simulink model "FOC_RL"  (R2023b)
settings: Solver=VariableStepAuto  StartTime=0.0  StopTime=30  RelTol=1e-3
InitFcn:
  | Resistencia = 0.679;
  | Inductancia = 0.01;
undefined symbols (not defined in the file): angulo, frac_polar, fuerza, magnitude
libraries: eeTransforms x3, slpidlib x3
settings Model: Creator=USUARIO  LastModifiedBy=USUARIO

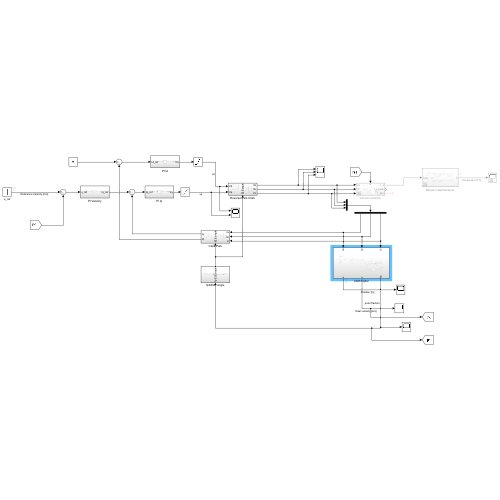
[thumbnail: Simulink's stored preview of the top-level diagram]
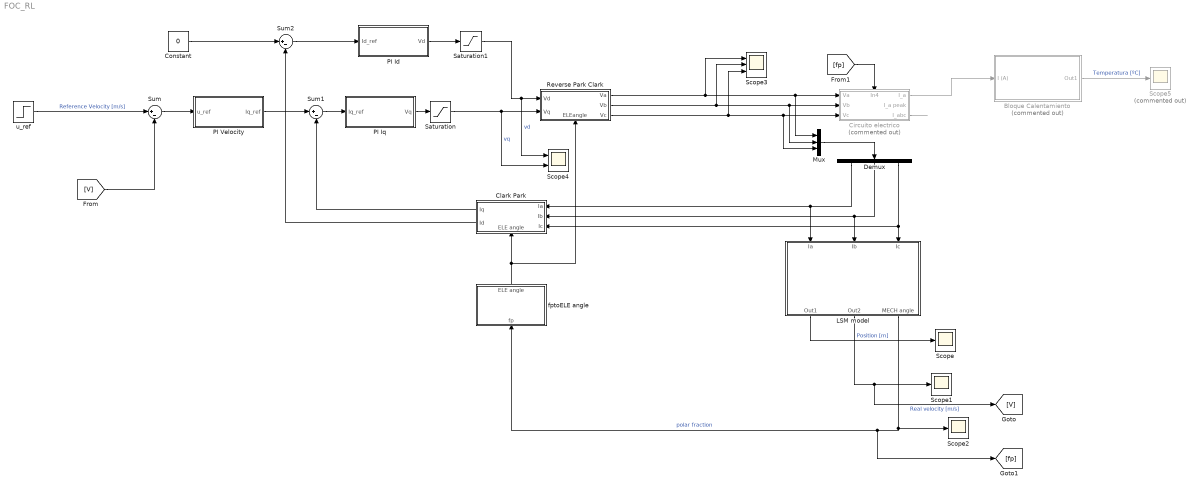
== system FOC_RL ==
  Bloque Calentamiento : Subsystem  Commented=on
  Circuito electrico : Subsystem  Commented=on
      settings: PortSchema="{\"entries\":[{\"content\":{\"sides\":[{\"content\":{\"connectorIds\":[\"In1\",\"In2\",\"In3\"]},\"type\":\"ConnectorPlacement.EquallySpacedRectSide\",\"uuid\":\"3f81a6db-fb69-453a-a09a-736cf4e6fbdf\"},{\"content\":{\"connectorIds\":[\"Out1\",\"Out2\",\"Out3\"],\"side\":\"RIGHT\"},\"type\":\"ConnectorPlacement.EquallySpacedRectSide\",\"uuid\":\"28f19065-0fce-4caf-9d5e-808d35e6acc4\"},{\"content\":{\"connectorIds\":[\"In4\"],\"side\":\"TOP\"},\"type\":\"ConnectorPlacement.EquallySpacedRectSide\",\"uuid\":\"0f0f3d94-64b2-4ad8-85c5-3a76de2037a2\"}]},\"type\":\"ConnectorPlacement.EquallySpacedConnector\",\"uuid\":\"ca84a14e-6f4b-4b2e-8a9f-b6683e76143b\"}],\"packageUris\":[\"http://schema.mathworks.com/mf0/Connector/R2020b\"],\"version\":\"1.0\"}"
  Clark Park : Subsystem
      settings: PortSchema="{\"entries\":[{\"content\":{\"sides\":[{\"content\":{\"connectorIds\":[\"Out1\",\"Out2\"]},\"type\":\"ConnectorPlacement.EquallySpacedRectSide\",\"uuid\":\"b73a0972-bf68-45ae-9239-d3343df02446\"},{\"content\":{\"connectorIds\":[\"In2\",\"In3\",\"In4\"],\"side\":\"RIGHT\"},\"type\":\"ConnectorPlacement.EquallySpacedRectSide\",\"uuid\":\"fec89271-c2ef-4885-992a-4c0db260d6e2\"},{\"content\":{\"side\":\"TOP\"},\"type\":\"ConnectorPlacement.EquallySpacedRectSide\",\"uuid\":\"51dbb3d3-34a9-43d7-9c98-9fa2f2011719\"},{\"content\":{\"connectorIds\":[\"In1\"],\"side\":\"BOTTOM\"},\"type\":\"ConnectorPlacement.EquallySpacedRectSide\",\"uuid\":\"eab6f42e-44ed-4b27-921c-43f03788cacc\"}]},\"type\":\"ConnectorPlacement.EquallySpacedConnector\",\"uuid\":\"a64495c7-a005-4dee-b109-5230f9247adc\"}],\"packageUris\":[\"http://schema.mathworks.com/mf0/Connector/R2020b\"],\"version\":\"1.0\"}"
  Constant : Constant  Value=0
  Demux : Demux  Outputs=3
  LSM model : Subsystem
      settings: PortSchema="{\"entries\":[{\"content\":{\"sides\":[{\"content\":{},\"type\":\"ConnectorPlacement.EquallySpacedRectSide\",\"uuid\":\"cac53d69-c428-44dc-bdf5-c688872b0596\"},{\"content\":{\"side\":\"RIGHT\"},\"type\":\"ConnectorPlacement.EquallySpacedRectSide\",\"uuid\":\"eab58244-5d35-448a-9540-885c93543b87\"},{\"content\":{\"connectorIds\":[\"In1\",\"In2\",\"In3\"],\"side\":\"TOP\"},\"type\":\"ConnectorPlacement.EquallySpacedRectSide\",\"uuid\":\"c64ce138-6960-4dd5-9e90-e1ffecc69b70\"},{\"content\":{\"connectorIds\":[\"Out1\",\"Out2\",\"Out3\"],\"side\":\"BOTTOM\"},\"type\":\"ConnectorPlacement.EquallySpacedRectSide\",\"uuid\":\"eda83129-b662-4da7-9603-68b1882420cc\"}]},\"type\":\"ConnectorPlacement.EquallySpacedConnector\",\"uuid\":\"82b650b8-86c6-4f03-ba07-634d14e4b94d\"}],\"packageUris\":[\"http://schema.mathworks.com/mf0/Connector/R2020b\"],\"version\":\"1.0\"}"
  Mux : Mux  Inputs=3
  PI Id : Subsystem
  PI Iq : Subsystem
  PI Velocity : Subsystem
  Reverse Park Clark : Subsystem
      settings: PortSchema="{\"entries\":[{\"content\":{\"sides\":[{\"content\":{\"connectorIds\":[\"In1\",\"In2\"]},\"type\":\"ConnectorPlacement.EquallySpacedRectSide\",\"uuid\":\"bb4b1d20-48ba-4b2f-b253-a250226ab501\"},{\"content\":{\"connectorIds\":[\"Out1\",\"Out2\",\"Out3\"],\"side\":\"RIGHT\"},\"type\":\"ConnectorPlacement.EquallySpacedRectSide\",\"uuid\":\"4768cfae-b67e-4820-9de3-2f5fe637e53a\"},{\"content\":{\"side\":\"TOP\"},\"type\":\"ConnectorPlacement.EquallySpacedRectSide\",\"uuid\":\"af639b0a-05db-45f8-bbbc-8f88455894ca\"},{\"content\":{\"connectorIds\":[\"In3\"],\"side\":\"BOTTOM\"},\"type\":\"ConnectorPlacement.EquallySpacedRectSide\",\"uuid\":\"149993ad-8fc7-43c9-baef-e4c40b0fb2ea\"}]},\"type\":\"ConnectorPlacement.EquallySpacedConnector\",\"uuid\":\"6dc62ad4-a38d-4494-a0f6-179f186f788d\"}],\"packageUris\":[\"http://schema.mathworks.com/mf0/Connector/R2020b\"],\"version\":\"1.0\"}"
  Saturation : Saturate  UpperLimit=100  LowerLimit=-100
  Saturation1 : Saturate  UpperLimit=100  LowerLimit=-100
  Scope : Scope
  Scope1 : Scope
  Scope2 : Scope
  Scope3 : Scope  NumInputPorts=3
  Scope4 : Scope  NumInputPorts=2
  Scope5 : Scope  Commented=on
  Sum : Sum  Inputs=|+-
  Sum1 : Sum  Inputs=|+-
  Sum2 : Sum  Inputs=|+-
  fptoELE angle : Subsystem
      settings: PortSchema="{\"entries\":[{\"content\":{\"sides\":[{\"content\":{},\"type\":\"ConnectorPlacement.EquallySpacedRectSide\",\"uuid\":\"b73a0972-bf68-45ae-9239-d3343df02446\"},{\"content\":{\"side\":\"RIGHT\"},\"type\":\"ConnectorPlacement.EquallySpacedRectSide\",\"uuid\":\"fec89271-c2ef-4885-992a-4c0db260d6e2\"},{\"content\":{\"connectorIds\":[\"Out1\"],\"side\":\"TOP\"},\"type\":\"ConnectorPlacement.EquallySpacedRectSide\",\"uuid\":\"51dbb3d3-34a9-43d7-9c98-9fa2f2011719\"},{\"content\":{\"connectorIds\":[\"In1\"],\"side\":\"BOTTOM\"},\"type\":\"ConnectorPlacement.EquallySpacedRectSide\",\"uuid\":\"4816d69c-9e54-4057-b439-390caef350ee\"}]},\"type\":\"ConnectorPlacement.EquallySpacedConnector\",\"uuid\":\"a64495c7-a005-4dee-b109-5230f9247adc\"}],\"packageUris\":[\"http://schema.mathworks.com/mf0/Connector/R2020b\"],\"version\":\"1.0\"}"
  u_ref : Step  Before=0.001  After=2  SampleTime=0
  wires:
  Constant/1 -> Sum2/1
  LSM model/3(MECH angle) -> [fp], fptoELE angle/1(fp), Scope2/1  "polar fraction"
  Clark Park/2(Id) -> Sum2/2
  Sum/1 -> PI Velocity/1(u_ref)
  fptoELE angle/1(ELE angle) -> Reverse Park Clark/3(ELEangle), Clark Park/1(ELE angle)
  Clark Park/1(Iq) -> Sum1/2
  PI Iq/1(Vq) -> Saturation/1
  Sum2/1 -> PI Id/1(Id_ref)
  Reverse Park Clark/3(Vc) -> Scope3/3, Mux/3, Circuito electrico/3(Vc)
  u_ref/1 -> Sum/1  "Reference Velocity [m/s]"
  Reverse Park Clark/2(Vb) -> Scope3/2, Mux/2, Circuito electrico/2(Vb)
  PI Id/1(Vd) -> Saturation1/1
  Reverse Park Clark/1(Va) -> Scope3/1, Mux/1, Circuito electrico/1(Va)
  Sum1/1 -> PI Iq/1(Iq_ref)
  LSM model/1(Out1) -> Scope/1  "Position [m]"
  LSM model/2(Out2) -> [V], Scope1/1  "Real velocity [m/s]"
  Saturation/1 -> Scope4/2, Reverse Park Clark/2(Vq)  "vq"
  Saturation1/1 -> Reverse Park Clark/1(Vd), Scope4/1  "vd"
  PI Velocity/1(Iq_ref) -> Sum1/1
  [V] -> Sum/2
  Bloque Calentamiento/1(Out1) -> Scope5/1  "Temperatura [ºC]"
  [fp] -> Circuito electrico/4(In4)
  Circuito electrico/3(I_abc) -> ?
  Circuito electrico/1(I_a) -> Bloque Calentamiento/1(I (A))
  Mux/1 -> Demux/1
  Demux/1 -> Clark Park/2(Ia), LSM model/1(Ia)
  Demux/2 -> Clark Park/3(Ib), LSM model/2(Ib)
  Demux/3 -> Clark Park/4(Ic), LSM model/3(Ic)

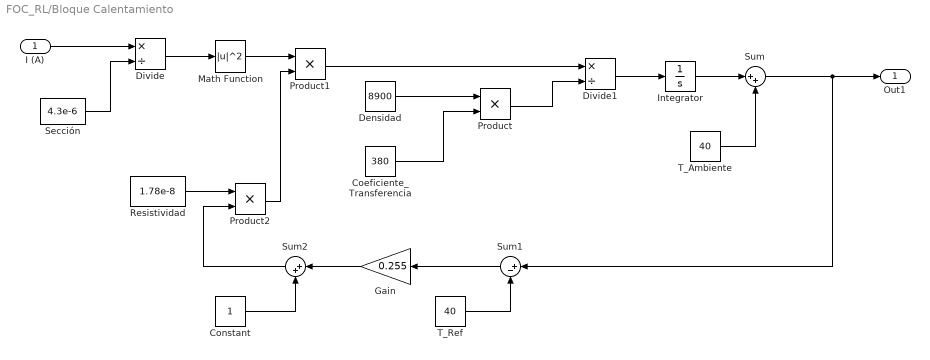
== system FOC_RL/Bloque Calentamiento ==
  I (A) : Inport
  Coeficiente_Transferencia : Constant  Value=380
  Constant : Constant
  Densidad : Constant  Value=8900
  Divide : Product  Inputs=*/
  Divide1 : Product  Inputs=*/
  Gain : Gain  Gain=0.255
  Integrator : Integrator
  Math Function : Math  Operator=magnitude^2
  Product : Product
  Product1 : Product
  Product2 : Product
  Resistividad : Constant  Value=1.78e-8
  Sección : Constant  Value=4.3e-6
  Sum : Sum  Inputs=|++
  Sum1 : Sum  Inputs=|+-
  Sum2 : Sum  Inputs=|++
  T_Ambiente : Constant  Value=40
  T_Ref : Constant  Value=40
  Out1 : Outport
  wires:
  I (A)/1 -> Divide/1
  Sección/1 -> Divide/2
  Divide/1 -> Math Function/1
  Densidad/1 -> Product/1
  Coeficiente_Transferencia/1 -> Product/2
  Product/1 -> Divide1/2
  Divide1/1 -> Integrator/1
  Math Function/1 -> Product1/1
  Product1/1 -> Divide1/1
  Resistividad/1 -> Product2/1
  Product2/1 -> Product1/2
  Integrator/1 -> Sum/1
  Sum/1 -> Sum1/1, Out1/1
  T_Ambiente/1 -> Sum/2
  Sum1/1 -> Gain/1
  T_Ref/1 -> Sum1/2
  Gain/1 -> Sum2/1
  Constant/1 -> Sum2/2
  Sum2/1 -> Product2/2

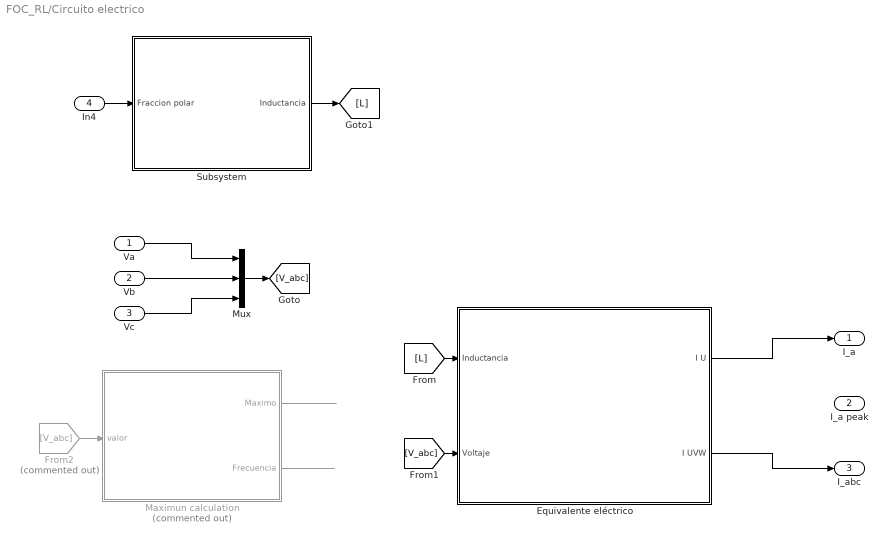
== system FOC_RL/Circuito electrico ==
  Va : Inport
  Vb : Inport  Port=2
  Vc : Inport  Port=3
  In4 : Inport  Port=4
  Equivalente eléctrico : Subsystem
  From2 : From  Commented=on  GotoTag=V_abc
  Maximun calculation : Subsystem  Commented=on
  Mux : Mux  Inputs=3
  Subsystem : Subsystem
  I_a : Outport
  I_a peak : Outport  Port=2
  I_abc : Outport  Port=3
  wires:
  Vc/1 -> Mux/3
  Vb/1 -> Mux/2
  Va/1 -> Mux/1
  Maximun calculation/2(Frecuencia) -> ?
  Maximun calculation/1(Maximo) -> ?
  Equivalente eléctrico/1(I U) -> I_a/1
  ? -> I_a peak/1
  Equivalente eléctrico/2(I UVW) -> I_abc/1
  Mux/1 -> [V_abc]
  Subsystem/1(Inductancia) -> [L]
  From2/1 -> Maximun calculation/1(valor)
  [V_abc] -> Equivalente eléctrico/2(Voltaje)
  [L] -> Equivalente eléctrico/1(Inductancia)
  In4/1 -> Subsystem/1(Fraccion polar)

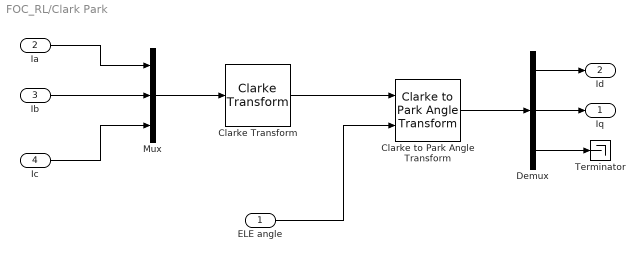
== system FOC_RL/Clark Park ==
  ELE angle : Inport
  Ia : Inport  Port=2
  Ib : Inport  Port=3
  Ic : Inport  Port=4
  Clarke Transform : eeTransforms/Clarke Transform  PowerInvariant=off
      settings: LibrarySourceBlock=|
      | ee_sl_lib/Mathematical
      | Transforms/Clarke Transform
  Clarke to Park Angle Transform : eeTransforms/Clarke to Park Angle Transform  AxisAlignment=Q-axis
      settings: LibrarySourceBlock=|
      | ee_sl_lib/Mathematical
      | Transforms/Clarke to Park
      | Angle Transform
  Demux : Demux  Outputs=3
  Mux : Mux  Inputs=3
  Terminator : Terminator
  Iq : Outport
  Id : Outport  Port=2
  wires:
  Ia/1 -> Mux/1
  Ib/1 -> Mux/2
  Ic/1 -> Mux/3
  Mux/1 -> Clarke Transform/1
  Clarke Transform/1 -> Clarke to Park Angle Transform/1
  ELE angle/1 -> Clarke to Park Angle Transform/2
  Clarke to Park Angle Transform/1 -> Demux/1
  Demux/1 -> Id/1
  Demux/2 -> Iq/1
  Demux/3 -> Terminator/1

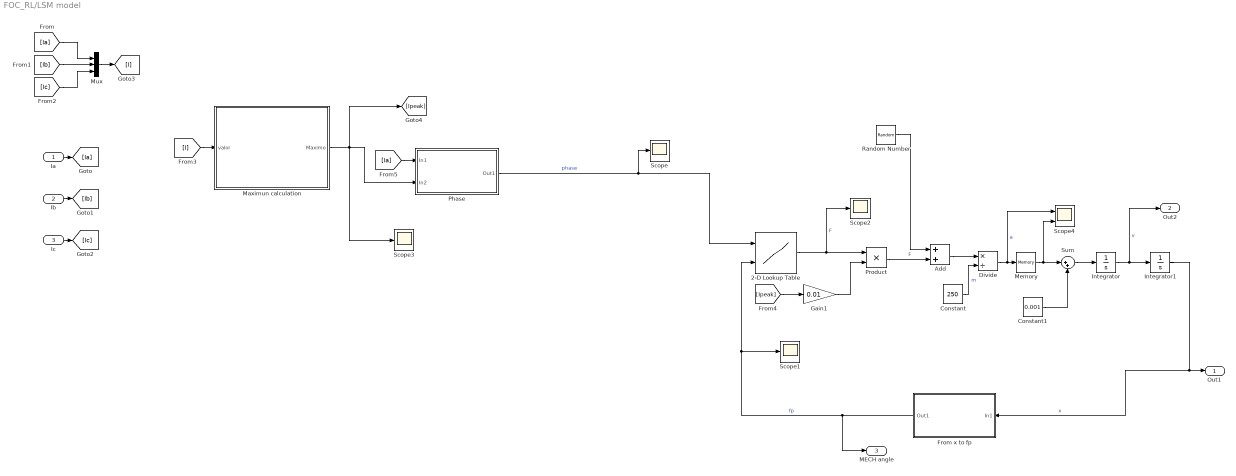
== system FOC_RL/LSM model ==
  Ia : Inport
  Ib : Inport  Port=2
  Ic : Inport  Port=3
  2-D Lookup Table : Lookup_n-D  BreakpointsForDimension1=angulo  BreakpointsForDimension2=frac_polar  Table=fuerza  InternalRulePriority=Speed  RndMeth=Simplest
      settings: InputPortMap=u0,u1
  Add : Sum
  Constant : Constant  Value=250
  Constant1 : Constant  Value=0.001
  Divide : Product  Inputs=*/
  From x to fp : Subsystem
  Gain1 : Gain  Gain=0.01
  Integrator : Integrator
  Integrator1 : Integrator
  Maximun calculation : Subsystem
  Memory : Memory
  Mux : Mux  Inputs=3
  Phase : Subsystem
  Product : Product
  Random Number : RandomNumber  Mean=-10  SampleTime=0.1
  Scope{,1..3} (4 alike) : Scope
  Scope4 : Scope  NumInputPorts=2
  Sum : Sum  Inputs=|++
  Out1 : Outport
  Out2 : Outport  Port=2
  MECH angle : Outport  Port=3
  wires:
  Product/1 -> Add/2  "F"
  Gain1/1 -> Product/2
  Maximun calculation/1(Maximo) -> [Ipeak], Scope3/1, Phase/2(In2)
  Add/1 -> Divide/1
  Random Number/1 -> Add/1
  Integrator/1 -> Out2/1, Integrator1/1  "v"
  Phase/1(Out1) -> Scope/1, 2-D Lookup Table/1  "phase"
  2-D Lookup Table/1 -> Scope2/1, Product/1  "F"
  Integrator1/1 -> From x to fp/1(In1), Out1/1  "x"
  Divide/1 -> Scope4/1, Memory/1  "a"
  From x to fp/1(Out1) -> MECH angle/1, Scope1/1, 2-D Lookup Table/2  "fp"
  Constant/1 -> Divide/2  "m"
  Ia/1 -> [Ia]
  Ic/1 -> [Ic]
  Ib/1 -> [Ib]
  [Ia] -> Mux/1
  [Ib] -> Mux/2
  [Ic] -> Mux/3
  Mux/1 -> [I]
  [I] -> Maximun calculation/1(valor)
  [Ipeak] -> Gain1/1
  [Ia] -> Phase/1(In1)
  Memory/1 -> Sum/1, Scope4/2
  Sum/1 -> Integrator/1
  Constant1/1 -> Sum/2

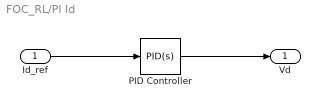
== system FOC_RL/PI Id ==
  Id_ref : Inport
  PID Controller : slpidlib/PID Controller  Controller=PID  Form=Parallel  TimeDomain=Continuous-time  UseExternalTs=off  SampleTime=-1  IntegratorMethod=Forward Euler  FilterMethod=Forward Euler  ControllerParametersSource=internal  P=1  I=1  UseKiTs=off  D=0  N=100  UseFilter=on  TunerSelectOption=Transfer Function Based (PID Tuner App)  InitialConditionSource=internal  InitialConditionForIntegrator=0  InitialConditionForFilter=0  DifferentiatorICPrevScaledInput=0  ExternalReset=none  TrackingMode=off  Kt=1  LimitOutput=off  SatLimitsSource=internal  UpperSaturationLimit=inf  LowerSaturationLimit=-inf  LinearizeAsGain=on  AntiWindupMode=none  Kb=1  LimitIntegrator=off  UpperIntegratorSaturationLimit=inf  LowerIntegratorSaturationLimit=-inf  POutMin=[]  POutMax=[]  IOutMin=[]  IOutMax=[]  DOutMin=[]  DOutMax=[]  NOutMin=[]  NOutMax=[]  SumOutMin=[]  SumOutMax=[]  SaturationOutMin=[]  SaturationOutMax=[]  PParamMin=[]  PParamMax=[]  IParamMin=[]  IParamMax=[]  DParamMin=[]  DParamMax=[]  NParamMin=[]  NParamMax=[]  KbParamMin=[]  KbParamMax=[]  KtParamMin=[]  KtParamMax=[]  KbOutMin=[]  KbOutMax=[]  KtOutMin=[]  KtOutMax=[]  IntegratorOutMin=[]  IntegratorOutMax=[]  FilterOutMin=[]  FilterOutMax=[]  SumI1OutMin=[]  SumI1OutMax=[]  SumI2OutMin=[]  SumI2OutMax=[]  SumI3OutMin=[]  SumI3OutMax=[]  SumI4OutMin=[]  SumI4OutMax=[]  SumDOutMin=[]  SumDOutMax=[]  DifferentiatorOutMin=[]  DifferentiatorOutMax=[]  FilterDiffOutCoefMin=[]  FilterDiffOutCoefMax=[]  ReciprocalOutMin=[]  ReciprocalOutMax=[]  SumDenOutMin=[]  SumDenOutMax=[]  SumNumOutMin=[]  SumNumOutMax=[]  DivideOutMin=[]  DivideOutMax=[]  UdiffTsProdOutMin=[]  UdiffTsProdOutMax=[]  NTsProdOutMin=[]  NTsProdOutMax=[]  UintegralTsProdOutMin=[]  UintegralTsProdOutMax=[]  UngainTsProdOutMin=[]  UngainTsProdOutMax=[]  ClampingZeroOutDataTypeStr=Inherit: Inherit via back propagation  ClampingZeroOutMin=[]  ClampingZeroOutMax=[]  FilterDenConstantOutDataTypeStr=Inherit: Inherit via back propagation  FilterDenConstantOutMin=[]  FilterDenConstantOutMax=[]  PCopyOutDataTypeStr=Inherit: Inherit via back propagation  PCopyOutMin=[]  PCopyOutMax=[]  NCopyOutDataTypeStr=Inherit: Inherit via back propagation  NCopyOutMin=[]  NCopyOutMax=[]  IntegratorContinuousStateAttributes=''  IntegratorStateMustResolveToSignalObject=off  IntegratorRTWStateStorageClass=Auto  FilterContinuousStateAttributes=''  FilterStateMustResolveToSignalObject=off  FilterRTWStateStorageClass=Auto  ParallelPVariant=InternalParameters  IdealPVariant=Disabled  IVariant=InternalParameters  DVariant=InternalParameters  IntegratorVariant=Continuous  SatVariant=Disabled  AWVariant=Passthrough  PCopyVariant=Disabled  TRVariant=Disabled  FdbkBlocksVariant=Forward  IdealPFdbkVariant=Disabled  SatFdbkVariant=Disabled  DerivativeFilterVariant=ContFilter  NVariant=InternalParameters  NCopyVariant=Disabled  FilterICVariant=InternalICsFilter  IntegratorICVariant=InternalICs  ExternalResetVariant=Disabled  TRSumVariant=Passthrough  SumFdbkVariant=Disabled  SumVariant=Sum_PID  TsampFilterVariant=InternalTs  TsampNgainVariant=Passthrough  TsampIntegralVariant=Disabled_SignalSpec  ExternalSaturationOutDataTypeStr=Inherit: Same as second input
  Vd : Outport
  wires:
  Id_ref/1 -> PID Controller/1
  PID Controller/1 -> Vd/1

== system FOC_RL/PI Iq ==
  Iq_ref : Inport
  PID Controller : slpidlib/PID Controller  Controller=PID  Form=Parallel  TimeDomain=Continuous-time  UseExternalTs=off  SampleTime=-1  IntegratorMethod=Forward Euler  FilterMethod=Forward Euler  ControllerParametersSource=internal  P=1  I=1  UseKiTs=off  D=0  N=100  UseFilter=on  TunerSelectOption=Transfer Function Based (PID Tuner App)  InitialConditionSource=internal  InitialConditionForIntegrator=0  InitialConditionForFilter=0  DifferentiatorICPrevScaledInput=0  ExternalReset=none  TrackingMode=off  Kt=1  LimitOutput=off  SatLimitsSource=internal  UpperSaturationLimit=inf  LowerSaturationLimit=-inf  LinearizeAsGain=on  AntiWindupMode=none  Kb=1  LimitIntegrator=off  UpperIntegratorSaturationLimit=inf  LowerIntegratorSaturationLimit=-inf  POutMin=[]  POutMax=[]  IOutMin=[]  IOutMax=[]  DOutMin=[]  DOutMax=[]  NOutMin=[]  NOutMax=[]  SumOutMin=[]  SumOutMax=[]  SaturationOutMin=[]  SaturationOutMax=[]  PParamMin=[]  PParamMax=[]  IParamMin=[]  IParamMax=[]  DParamMin=[]  DParamMax=[]  NParamMin=[]  NParamMax=[]  KbParamMin=[]  KbParamMax=[]  KtParamMin=[]  KtParamMax=[]  KbOutMin=[]  KbOutMax=[]  KtOutMin=[]  KtOutMax=[]  IntegratorOutMin=[]  IntegratorOutMax=[]  FilterOutMin=[]  FilterOutMax=[]  SumI1OutMin=[]  SumI1OutMax=[]  SumI2OutMin=[]  SumI2OutMax=[]  SumI3OutMin=[]  SumI3OutMax=[]  SumI4OutMin=[]  SumI4OutMax=[]  SumDOutMin=[]  SumDOutMax=[]  DifferentiatorOutMin=[]  DifferentiatorOutMax=[]  FilterDiffOutCoefMin=[]  FilterDiffOutCoefMax=[]  ReciprocalOutMin=[]  ReciprocalOutMax=[]  SumDenOutMin=[]  SumDenOutMax=[]  SumNumOutMin=[]  SumNumOutMax=[]  DivideOutMin=[]  DivideOutMax=[]  UdiffTsProdOutMin=[]  UdiffTsProdOutMax=[]  NTsProdOutMin=[]  NTsProdOutMax=[]  UintegralTsProdOutMin=[]  UintegralTsProdOutMax=[]  UngainTsProdOutMin=[]  UngainTsProdOutMax=[]  ClampingZeroOutDataTypeStr=Inherit: Inherit via back propagation  ClampingZeroOutMin=[]  ClampingZeroOutMax=[]  FilterDenConstantOutDataTypeStr=Inherit: Inherit via back propagation  FilterDenConstantOutMin=[]  FilterDenConstantOutMax=[]  PCopyOutDataTypeStr=Inherit: Inherit via back propagation  PCopyOutMin=[]  PCopyOutMax=[]  NCopyOutDataTypeStr=Inherit: Inherit via back propagation  NCopyOutMin=[]  NCopyOutMax=[]  IntegratorContinuousStateAttributes=''  IntegratorStateMustResolveToSignalObject=off  IntegratorRTWStateStorageClass=Auto  FilterContinuousStateAttributes=''  FilterStateMustResolveToSignalObject=off  FilterRTWStateStorageClass=Auto  ParallelPVariant=InternalParameters  IdealPVariant=Disabled  IVariant=InternalParameters  DVariant=InternalParameters  IntegratorVariant=Continuous  SatVariant=Disabled  AWVariant=Passthrough  PCopyVariant=Disabled  TRVariant=Disabled  FdbkBlocksVariant=Forward  IdealPFdbkVariant=Disabled  SatFdbkVariant=Disabled  DerivativeFilterVariant=ContFilter  NVariant=InternalParameters  NCopyVariant=Disabled  FilterICVariant=InternalICsFilter  IntegratorICVariant=InternalICs  ExternalResetVariant=Disabled  TRSumVariant=Passthrough  SumFdbkVariant=Disabled  SumVariant=Sum_PID  TsampFilterVariant=InternalTs  TsampNgainVariant=Passthrough  TsampIntegralVariant=Disabled_SignalSpec  ExternalSaturationOutDataTypeStr=Inherit: Same as second input
  Vq : Outport
  wires:
  Iq_ref/1 -> PID Controller/1
  PID Controller/1 -> Vq/1

== system FOC_RL/PI Velocity ==
  u_ref : Inport
  PID Controller : slpidlib/PID Controller  Controller=PID  Form=Parallel  TimeDomain=Continuous-time  UseExternalTs=off  SampleTime=-1  IntegratorMethod=Forward Euler  FilterMethod=Forward Euler  ControllerParametersSource=internal  P=50  I=5  UseKiTs=off  D=0  N=100  UseFilter=on  TunerSelectOption=Transfer Function Based (PID Tuner App)  InitialConditionSource=internal  InitialConditionForIntegrator=0  InitialConditionForFilter=0  DifferentiatorICPrevScaledInput=0  ExternalReset=none  TrackingMode=off  Kt=1  LimitOutput=off  SatLimitsSource=internal  UpperSaturationLimit=inf  LowerSaturationLimit=-inf  LinearizeAsGain=on  AntiWindupMode=none  Kb=1  LimitIntegrator=off  UpperIntegratorSaturationLimit=inf  LowerIntegratorSaturationLimit=-inf  POutMin=[]  POutMax=[]  IOutMin=[]  IOutMax=[]  DOutMin=[]  DOutMax=[]  NOutMin=[]  NOutMax=[]  SumOutMin=[]  SumOutMax=[]  SaturationOutMin=[]  SaturationOutMax=[]  PParamMin=[]  PParamMax=[]  IParamMin=[]  IParamMax=[]  DParamMin=[]  DParamMax=[]  NParamMin=[]  NParamMax=[]  KbParamMin=[]  KbParamMax=[]  KtParamMin=[]  KtParamMax=[]  KbOutMin=[]  KbOutMax=[]  KtOutMin=[]  KtOutMax=[]  IntegratorOutMin=[]  IntegratorOutMax=[]  FilterOutMin=[]  FilterOutMax=[]  SumI1OutMin=[]  SumI1OutMax=[]  SumI2OutMin=[]  SumI2OutMax=[]  SumI3OutMin=[]  SumI3OutMax=[]  SumI4OutMin=[]  SumI4OutMax=[]  SumDOutMin=[]  SumDOutMax=[]  DifferentiatorOutMin=[]  DifferentiatorOutMax=[]  FilterDiffOutCoefMin=[]  FilterDiffOutCoefMax=[]  ReciprocalOutMin=[]  ReciprocalOutMax=[]  SumDenOutMin=[]  SumDenOutMax=[]  SumNumOutMin=[]  SumNumOutMax=[]  DivideOutMin=[]  DivideOutMax=[]  UdiffTsProdOutMin=[]  UdiffTsProdOutMax=[]  NTsProdOutMin=[]  NTsProdOutMax=[]  UintegralTsProdOutMin=[]  UintegralTsProdOutMax=[]  UngainTsProdOutMin=[]  UngainTsProdOutMax=[]  ClampingZeroOutDataTypeStr=Inherit: Inherit via back propagation  ClampingZeroOutMin=[]  ClampingZeroOutMax=[]  FilterDenConstantOutDataTypeStr=Inherit: Inherit via back propagation  FilterDenConstantOutMin=[]  FilterDenConstantOutMax=[]  PCopyOutDataTypeStr=Inherit: Inherit via back propagation  PCopyOutMin=[]  PCopyOutMax=[]  NCopyOutDataTypeStr=Inherit: Inherit via back propagation  NCopyOutMin=[]  NCopyOutMax=[]  IntegratorContinuousStateAttributes=''  IntegratorStateMustResolveToSignalObject=off  IntegratorRTWStateStorageClass=Auto  FilterContinuousStateAttributes=''  FilterStateMustResolveToSignalObject=off  FilterRTWStateStorageClass=Auto  ParallelPVariant=InternalParameters  IdealPVariant=Disabled  IVariant=InternalParameters  DVariant=InternalParameters  IntegratorVariant=Continuous  SatVariant=Disabled  AWVariant=Passthrough  PCopyVariant=Disabled  TRVariant=Disabled  FdbkBlocksVariant=Forward  IdealPFdbkVariant=Disabled  SatFdbkVariant=Disabled  DerivativeFilterVariant=ContFilter  NVariant=InternalParameters  NCopyVariant=Disabled  FilterICVariant=InternalICsFilter  IntegratorICVariant=InternalICs  ExternalResetVariant=Disabled  TRSumVariant=Passthrough  SumFdbkVariant=Disabled  SumVariant=Sum_PID  TsampFilterVariant=InternalTs  TsampNgainVariant=Passthrough  TsampIntegralVariant=Disabled_SignalSpec  ExternalSaturationOutDataTypeStr=Inherit: Same as second input
  Iq_ref : Outport
  wires:
  u_ref/1 -> PID Controller/1
  PID Controller/1 -> Iq_ref/1

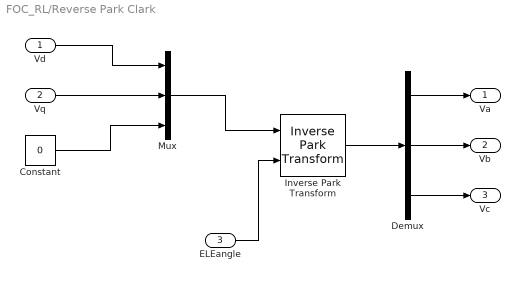
== system FOC_RL/Reverse Park Clark ==
  Vd : Inport
  Vq : Inport  Port=2
  ELEangle : Inport  Port=3
  Constant : Constant  Value=0
  Demux : Demux  Outputs=3
  Inverse Park Transform : eeTransforms/Inverse Park Transform  AxisAlignment=Q-axis  PowerInvariant=off
      settings: LibrarySourceBlock=|
      | ee_sl_lib/Mathematical
      | Transforms/Inverse
      | Park Transform
  Mux : Mux  Inputs=3
  Va : Outport
  Vb : Outport  Port=2
  Vc : Outport  Port=3
  wires:
  Demux/1 -> Va/1
  Demux/2 -> Vb/1
  Demux/3 -> Vc/1
  Inverse Park Transform/1 -> Demux/1
  Vd/1 -> Mux/1
  Vq/1 -> Mux/2
  Constant/1 -> Mux/3
  Mux/1 -> Inverse Park Transform/1
  ELEangle/1 -> Inverse Park Transform/2

== system FOC_RL/fptoELE angle ==
  fp : Inport
  Gain : Gain  Gain=pi
  ELE angle : Outport
  wires:
  fp/1 -> Gain/1
  Gain/1 -> ELE angle/1

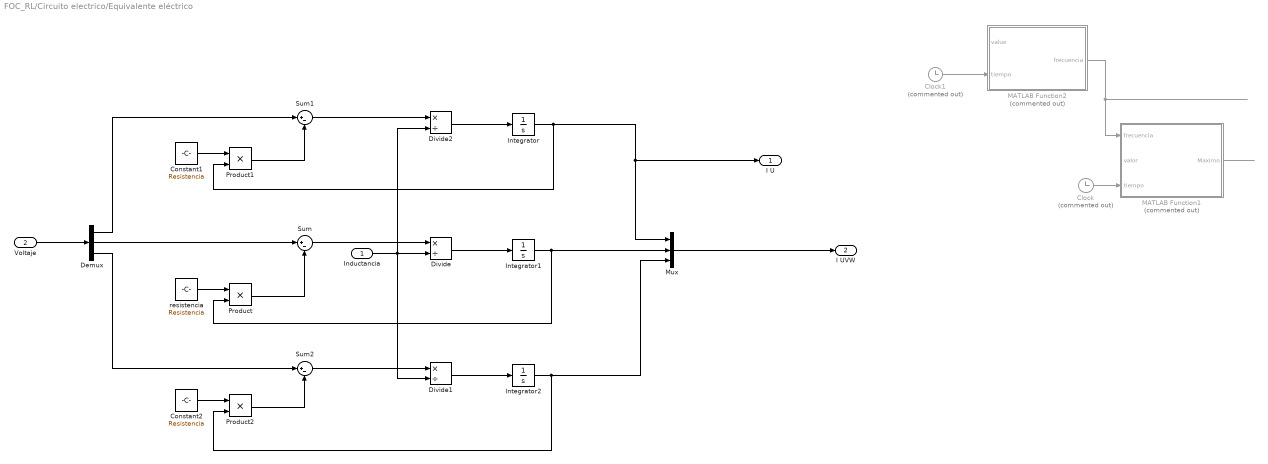
== system FOC_RL/Circuito electrico/Equivalente eléctrico ==
  Inductancia : Inport
  Voltaje : Inport  Port=2
  Clock : Clock  Commented=on
  Clock1 : Clock  Commented=on
  Constant1 : Constant  Value=Resistencia
  Constant2 : Constant  Value=Resistencia
  Demux : Demux  Outputs=3
  Divide : Product  Inputs=*/
  Divide1 : Product  Inputs=*/
  Divide2 : Product  Inputs=*/
  Integrator : Integrator
  Integrator1 : Integrator
  Integrator2 : Integrator
  MATLAB Function1 : MATLAB Function  Commented=on  TreatAsAtomicUnit=on
  MATLAB Function2 : MATLAB Function  Commented=on  TreatAsAtomicUnit=on
  Mux : Mux  Inputs=3
  Product : Product
  Product1 : Product
  Product2 : Product
  Sum : Sum  Inputs=|+-
  Sum1 : Sum  Inputs=|+-
  Sum2 : Sum  Inputs=|+-
  resistencia : Constant  Value=Resistencia
  I U : Outport
  I UVW : Outport  Port=2
  wires:
  Voltaje/1 -> Demux/1
  Demux/2 -> Sum/1
  Product/1 -> Sum/2
  resistencia/1 -> Product/1
  Sum/1 -> Divide/1
  Inductancia/1 -> Divide1/2, Divide2/2, Divide/2
  Product1/1 -> Sum1/2
  Sum1/1 -> Divide2/1
  Demux/1 -> Sum1/1
  Constant1/1 -> Product1/1
  Product2/1 -> Sum2/2
  Sum2/1 -> Divide1/1
  Demux/3 -> Sum2/1
  Constant2/1 -> Product2/1
  Divide2/1 -> Integrator/1
  Integrator/1 -> Product1/2, Mux/1, I U/1
  Divide/1 -> Integrator1/1
  Divide1/1 -> Integrator2/1
  Integrator1/1 -> Product/2, Mux/2
  Integrator2/1 -> Product2/2, Mux/3
  Mux/1 -> I UVW/1
  MATLAB Function1/1(Maximo) -> ?
  MATLAB Function2/1(frecuencia) -> MATLAB Function1/1(frecuencia)
  Clock/1 -> MATLAB Function1/3(tiempo)
  ? -> MATLAB Function2/1(value), MATLAB Function1/2(valor)
  Clock1/1 -> MATLAB Function2/2(tiempo)

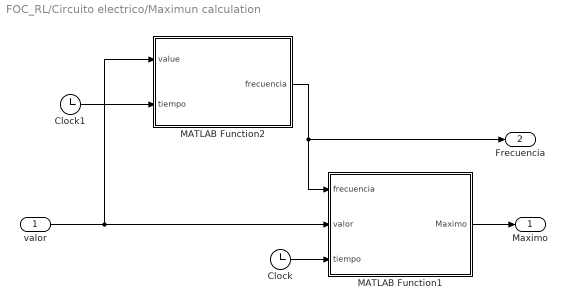
== system FOC_RL/Circuito electrico/Maximun calculation ==
  valor : Inport
  Clock : Clock
  Clock1 : Clock
  MATLAB Function1 : MATLAB Function  TreatAsAtomicUnit=on
  MATLAB Function2 : MATLAB Function  TreatAsAtomicUnit=on
  Maximo : Outport
  Frecuencia : Outport  Port=2
  wires:
  valor/1 -> MATLAB Function2/1(value), MATLAB Function1/2(valor)
  Clock/1 -> MATLAB Function1/3(tiempo)
  MATLAB Function2/1(frecuencia) -> Frecuencia/1, MATLAB Function1/1(frecuencia)
  Clock1/1 -> MATLAB Function2/2(tiempo)
  MATLAB Function1/1(Maximo) -> Maximo/1

== system FOC_RL/Circuito electrico/Subsystem ==
  Fraccion polar : Inport
  Constant : Constant  Value=Inductancia
  Inductancia : Outport
  wires:
  Fraccion polar/1 -> ?
  Constant/1 -> Inductancia/1

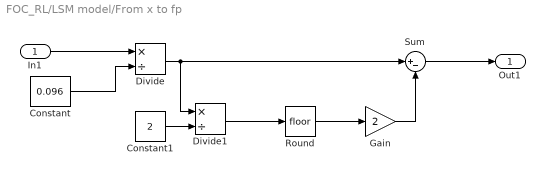
== system FOC_RL/LSM model/From x to fp ==
  In1 : Inport
  Constant : Constant  Value=0.096
  Constant1 : Constant  Value=2
  Divide : Product  Inputs=*/
  Divide1 : Product  Inputs=*/
  Gain : Gain  Gain=2
  Round : Rounding
  Sum : Sum  Inputs=|+-
  Out1 : Outport
  wires:
  In1/1 -> Divide/1
  Constant/1 -> Divide/2
  Divide/1 -> Divide1/1, Sum/1
  Divide1/1 -> Round/1
  Round/1 -> Gain/1
  Constant1/1 -> Divide1/2
  Gain/1 -> Sum/2
  Sum/1 -> Out1/1

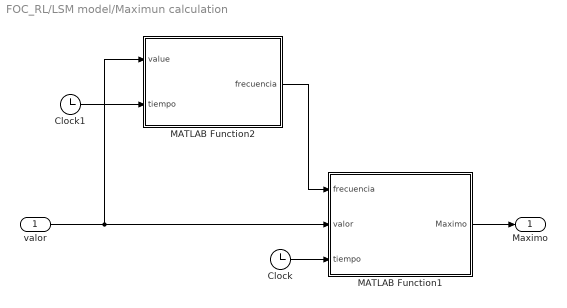
== system FOC_RL/LSM model/Maximun calculation ==
  valor : Inport
  Clock : Clock
  Clock1 : Clock
  MATLAB Function1 : MATLAB Function  TreatAsAtomicUnit=on
  MATLAB Function2 : MATLAB Function  TreatAsAtomicUnit=on
  Maximo : Outport
  wires:
  valor/1 -> MATLAB Function2/1(value), MATLAB Function1/2(valor)
  Clock/1 -> MATLAB Function1/3(tiempo)
  MATLAB Function2/1(frecuencia) -> MATLAB Function1/1(frecuencia)
  Clock1/1 -> MATLAB Function2/2(tiempo)
  MATLAB Function1/1(Maximo) -> Maximo/1

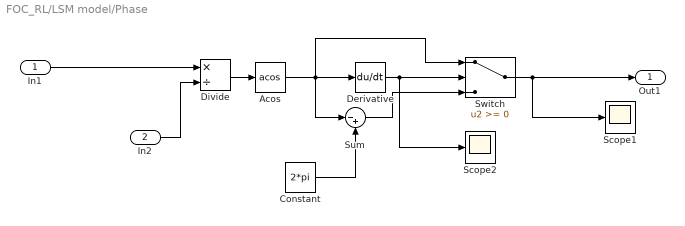
== system FOC_RL/LSM model/Phase ==
  In1 : Inport
  In2 : Inport  Port=2
  Acos : Trigonometry  Operator=acos
  Constant : Constant  Value=2*pi
  Derivative : Derivative
  Divide : Product  Inputs=*/
  Scope1 : Scope
  Scope2 : Scope
  Sum : Sum  Inputs=|-+
  Switch : Switch  SaturateOnIntegerOverflow=off  InputSameDT=off
  Out1 : Outport
  wires:
  In1/1 -> Divide/1
  Derivative/1 -> Scope2/1, Switch/2
  Acos/1 -> Switch/1, Sum/1, Derivative/1
  Sum/1 -> Switch/3
  Switch/1 -> Out1/1, Scope1/1
  Constant/1 -> Sum/2
  In2/1 -> Divide/2
  Divide/1 -> Acos/1

== matlab function FOC_RL/LSM model/Maximun calculation/MATLAB Function1 ==
  settings: updateMethod=DISCRETE
  data: frecuencia input; Maximo output; valor input; tiempo input
function Maximo = fcn(frecuencia,valor,tiempo)

   persistent antiguo_maximo
    if isempty(antiguo_maximo)
       antiguo_maximo=0;
    end
    persistent t_maximo
    if isempty(t_maximo)
       t_maximo=0;
    end

maximo = [0 0 0];

periodo=1/abs(frecuencia)/3;

for i=1:3
    if abs(valor(i))>=antiguo_maximo
        maximo(i)=abs(valor(i));
        antiguo_maximo=abs(valor(i));
        t_maximo=tiempo;
    else
        maximo(i)=antiguo_maximo;
        if tiempo>t_maximo+periodo
            maximo(i)=abs(valor(i));
            antiguo_maximo=abs(valor(i));
            t_maximo=tiempo;
        end
    end
end

Maximo = max(maximo);

== matlab function FOC_RL/LSM model/Maximun calculation/MATLAB Function2 ==
  settings: updateMethod=DISCRETE
  data: frecuencia output; value input; tiempo input
function frecuencia = frecuency_calculator(value,tiempo)

   persistent signo
    if isempty(signo)
       signo=[0 0 0]; % 1 positive, 2 negative
    end
    persistent t_inicio
    if isempty(t_inicio)
       t_inicio=[0 0 0];
    end

    persistent frecuencia_acc
    if isempty(frecuencia_acc)
       frecuencia_acc=1;
    end

    frecuencia=frecuencia_acc;

    for i=1:3
    
        if signo(i) == 0
            if value(i) >= 0 
                signo(i) = 1;
            else
                signo(i) = 2;
            end
            t_inicio(i)=tiempo;
        end
        
        if signo(i)==1
            if value(i) <= 0
                frecuencia = 1/(2*(tiempo-t_inicio(i)));
                frecuencia_acc=frecuencia;
                signo(i) = 0;
            end
        end
        
        if signo(i)==2
            if value(i) >= 0
                frecuencia = 1/(2*(tiempo-t_inicio(i)));
                frecuencia_acc=frecuencia;
                signo(i) = 0;
            end
        end

    end

== matlab function FOC_RL/Circuito electrico/Maximun calculation/MATLAB Function1 ==
  settings: updateMethod=DISCRETE
  data: frecuencia input; Maximo output; valor input; tiempo input
function Maximo = fcn(frecuencia,valor,tiempo)

   persistent antiguo_maximo
    if isempty(antiguo_maximo)
       antiguo_maximo=0;
    end
    persistent t_maximo
    if isempty(t_maximo)
       t_maximo=0;
    end

maximo = [0 0 0];

periodo=1/abs(frecuencia)/3;

for i=1:3
    if abs(valor(i))>=antiguo_maximo
        maximo(i)=abs(valor(i));
        antiguo_maximo=abs(valor(i));
        t_maximo=tiempo;
    else
        maximo(i)=antiguo_maximo;
        if tiempo>t_maximo+periodo
            maximo(i)=abs(valor(i));
            antiguo_maximo=abs(valor(i));
            t_maximo=tiempo;
        end
    end
end

Maximo = max(maximo);

== matlab function FOC_RL/Circuito electrico/Maximun calculation/MATLAB Function2 ==
  settings: updateMethod=DISCRETE
  data: frecuencia output; value input; tiempo input
function frecuencia = frecuency_calculator(value,tiempo)

   persistent signo
    if isempty(signo)
       signo=[0 0 0]; % 1 positive, 2 negative
    end
    persistent t_inicio
    if isempty(t_inicio)
       t_inicio=[0 0 0];
    end

    persistent frecuencia_acc
    if isempty(frecuencia_acc)
       frecuencia_acc=1;
    end

    frecuencia=frecuencia_acc;

    for i=1:3
    
        if signo(i) == 0
            if value(i) >= 0 
                signo(i) = 1;
            else
                signo(i) = 2;
            end
            t_inicio(i)=tiempo;
        end
        
        if signo(i)==1
            if value(i) <= 0
                frecuencia = 1/(2*(tiempo-t_inicio(i)));
                frecuencia_acc=frecuencia;
                signo(i) = 0;
            end
        end
        
        if signo(i)==2
            if value(i) >= 0
                frecuencia = 1/(2*(tiempo-t_inicio(i)));
                frecuencia_acc=frecuencia;
                signo(i) = 0;
            end
        end

    end

== matlab function FOC_RL/Circuito electrico/Equivalente eléctrico/MATLAB Function1 ==
  settings: updateMethod=DISCRETE
  data: frecuencia input; Maximo output; valor input; tiempo input
function Maximo = fcn(frecuencia,valor,tiempo)

   persistent antiguo_maximo
    if isempty(antiguo_maximo)
       antiguo_maximo=0;
    end
    persistent t_maximo
    if isempty(t_maximo)
       t_maximo=0;
    end

maximo = [0 0 0];

periodo=1/abs(frecuencia)/3;

for i=1:3
    if abs(valor(i))>=antiguo_maximo
        maximo(i)=abs(valor(i));
        antiguo_maximo=abs(valor(i));
        t_maximo=tiempo;
    else
        maximo(i)=antiguo_maximo;
        if tiempo>t_maximo+periodo
            maximo(i)=abs(valor(i));
            antiguo_maximo=abs(valor(i));
            t_maximo=tiempo;
        end
    end
end

Maximo = max(maximo);

== matlab function FOC_RL/Circuito electrico/Equivalente eléctrico/MATLAB Function2 ==
  settings: updateMethod=DISCRETE
  data: frecuencia output; value input; tiempo input
function frecuencia = frecuency_calculator(value,tiempo)

   persistent signo
    if isempty(signo)
       signo=[0 0 0]; % 1 positive, 2 negative
    end
    persistent t_inicio
    if isempty(t_inicio)
       t_inicio=[0 0 0];
    end

    persistent frecuencia_acc
    if isempty(frecuencia_acc)
       frecuencia_acc=1;
    end

    frecuencia=frecuencia_acc;

    for i=1:3
    
        if signo(i) == 0
            if value(i) >= 0 
                signo(i) = 1;
            else
                signo(i) = 2;
            end
            t_inicio(i)=tiempo;
        end
        
        if signo(i)==1
            if value(i) <= 0
                frecuencia = 1/(2*(tiempo-t_inicio(i)));
                frecuencia_acc=frecuencia;
                signo(i) = 0;
            end
        end
        
        if signo(i)==2
            if value(i) >= 0
                frecuencia = 1/(2*(tiempo-t_inicio(i)));
                frecuencia_acc=frecuencia;
                signo(i) = 0;
            end
        end

    end
